simulink model "rzad10"  (Simulink 7.9)
settings: Solver=ode4  StartTime=0.0  StopTime=5  FixedStep=0.01  RelTol=1e-3
values from neighbouring files (symbols this model uses):
  a = X0(2)    [pade_err.m]    (also in scr.m = 0.3826)
  b = X0(3)    [pade_err.m]    (also in scr.m = 1.0318)
undefined symbols (not defined in the file or in its folder): licz, mian
settings Model: Creator=student  LastModifiedBy=student

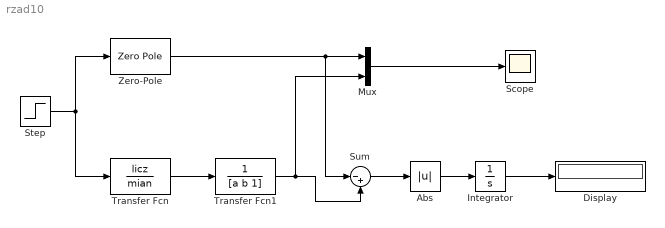
== system rzad10 ==
  Abs : Abs
  Display : Display
  Integrator : Integrator
  Mux : Mux  Inputs=2
  Scope : Scope
  Step : Step  Time=0  SampleTime=0
  Sum : Sum  Inputs=|-+
  Transfer Fcn : TransferFcn  Numerator=licz  Denominator=mian
  Transfer Fcn1 : TransferFcn  Denominator=[a b 1]
  Zero-Pole : ZeroPole  Zeros=[]  Poles=[-5 -5 -5 -5 -5 -5 -5 -5 -5 -5 ]  Gain=[5^10]
  wires:
  Step/1 -> Zero-Pole/1, Transfer Fcn/1
  Transfer Fcn/1 -> Transfer Fcn1/1
  Zero-Pole/1 -> Mux/1, Sum/1
  Transfer Fcn1/1 -> Sum/2, Mux/2
  Mux/1 -> Scope/1
  Sum/1 -> Abs/1
  Abs/1 -> Integrator/1
  Integrator/1 -> Display/1
